simulink model "ipad2"  (Simulink 7.8)
settings: Solver=ode23tb  StartTime=0.0  StopTime=0.2  RelTol=1e-4
libraries: powerlib x97, powerlib_extras x1
settings Model: Creator=srujana  LastModifiedBy=srujana
settings SolverCC: MaxConsecutiveMinStep=auto  SolverResetMethod=Robust

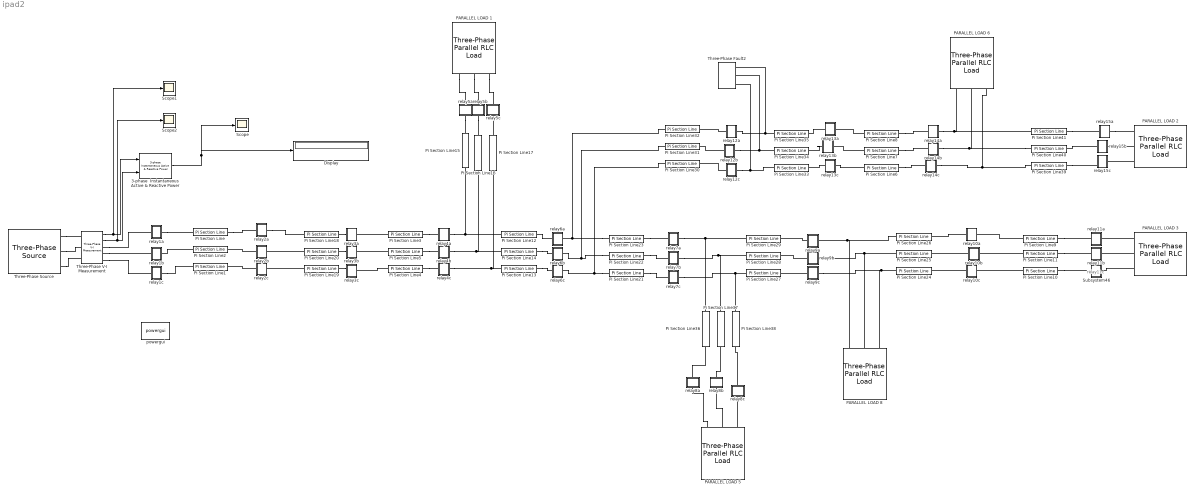
== system ipad2 ==
  note: relay11c
  3-phase  Instantaneous  Active & Reactive Power : powerlib_extras/Measurements/3-phase  Instantaneous  Active & Reactive Power
  Display : Display
      settings: Format=decimal (Stored Integer)
  PARALLEL LOAD 1 : powerlib/Elements/Three-Phase Parallel RLC Load  LConnTagsString=A|B|C  Configuration=Y (grounded)  NominalVoltage=10.27e3  NominalFrequency=50  ActivePower=1.85e6  InductivePower=1.28e6  CapacitivePower=0  Measurements=None  LoadType=constant Z
  PARALLEL LOAD 2 : powerlib/Elements/Three-Phase Parallel RLC Load  LConnTagsString=A|B|C  Configuration=Y (grounded)  NominalVoltage=10.27e3  NominalFrequency=50  ActivePower=0.91e6  InductivePower=0.63518e6  CapacitivePower=0  Measurements=None  LoadType=constant Z
  PARALLEL LOAD 3 : powerlib/Elements/Three-Phase Parallel RLC Load  LConnTagsString=A|B|C  Configuration=Y (grounded)  NominalVoltage=10.27e3  NominalFrequency=50  ActivePower=0.857e6  InductivePower=0.598e6  CapacitivePower=0  Measurements=None  LoadType=constant Z
  PARALLEL LOAD 5 : powerlib/Elements/Three-Phase Parallel RLC Load  LConnTagsString=A|B|C  Configuration=Y (grounded)  NominalVoltage=10.27e3  NominalFrequency=50  ActivePower=0.901e6  InductivePower=0.58046e6  CapacitivePower=0  Measurements=None  LoadType=constant Z
  PARALLEL LOAD 6 : powerlib/Elements/Three-Phase Parallel RLC Load  LConnTagsString=A|B|C  Configuration=Y (grounded)  NominalVoltage=10.27e3  NominalFrequency=50  ActivePower=0.92e6  InductivePower=0.64213e6  CapacitivePower=0  Measurements=None  LoadType=constant Z
  PARALLEL LOAD 8 : powerlib/Elements/Three-Phase Parallel RLC Load  LConnTagsString=A|B|C  Configuration=Y (grounded)  NominalVoltage=10.27e3  NominalFrequency=50  ActivePower=0.9e6  InductivePower=1.09756e6  CapacitivePower=0  Measurements=None  LoadType=constant Z
  Pi Section Line : powerlib/Elements/Pi Section Line  LConnTagsString=__new0  RConnTagsString=__new0  Frequency=50  Resistance=0.163  Inductance=0.28329e-3  Capacitance=445.633e-9  Length=0.078  PiSections=1  Measurements=None
      settings: AttributesFormatString=\n
  Pi Section Line1 : powerlib/Elements/Pi Section Line  LConnTagsString=__new0  RConnTagsString=__new0  Frequency=50  Resistance=0.163  Inductance=0.28329e-3  Capacitance=445.633e-9  Length=0.078  PiSections=1  Measurements=None
      settings: AttributesFormatString=\n
  Pi Section Line10 : powerlib/Elements/Pi Section Line  LConnTagsString=__new0  RConnTagsString=__new0  Frequency=50  Resistance=1.113  Inductance=0.37242e-3  Capacitance=190.985e-9  Length=0.1  PiSections=1  Measurements=None
      settings: AttributesFormatString=\n
  Pi Section Line11 : powerlib/Elements/Pi Section Line  LConnTagsString=__new0  RConnTagsString=__new0  Frequency=50  Resistance=1.113  Inductance=0.37242e-3  Capacitance=190.985e-9  Length=0.1  PiSections=1  Measurements=None
      settings: AttributesFormatString=\n
  Pi Section Line12 : powerlib/Elements/Pi Section Line  LConnTagsString=__new0  RConnTagsString=__new0  Frequency=50  Resistance=0.569  Inductance=0.3374e-3  Capacitance=254.647e-9  Length=0.33  PiSections=1  Measurements=None
      settings: AttributesFormatString=\n
  Pi Section Line13 : powerlib/Elements/Pi Section Line  LConnTagsString=__new0  RConnTagsString=__new0  Frequency=50  Resistance=0.569  Inductance=0.3374e-3  Capacitance=254.647e-9  Length=0.33  PiSections=1  Measurements=None
      settings: AttributesFormatString=\n
  Pi Section Line14 : powerlib/Elements/Pi Section Line  LConnTagsString=__new0  RConnTagsString=__new0  Frequency=50  Resistance=0.569  Inductance=0.3374e-3  Capacitance=254.647e-9  Length=0.33  PiSections=1  Measurements=None
      settings: AttributesFormatString=\n
  Pi Section Line15 : powerlib/Elements/Pi Section Line  LConnTagsString=__new0  RConnTagsString=__new0  Frequency=50  Resistance=0.569  Inductance=0.3374e-3  Capacitance=254.647e-9  Length=0.05  PiSections=1  Measurements=None
      settings: AttributesFormatString=\n
  Pi Section Line16 : powerlib/Elements/Pi Section Line  LConnTagsString=__new0  RConnTagsString=__new0  Frequency=50  Resistance=0.569  Inductance=0.3374e-3  Capacitance=254.647e-9  Length=0.05  PiSections=1  Measurements=None
      settings: AttributesFormatString=\n
  Pi Section Line17 : powerlib/Elements/Pi Section Line  LConnTagsString=__new0  RConnTagsString=__new0  Frequency=50  Resistance=0.569  Inductance=0.3374e-3  Capacitance=254.647e-9  Length=0.05  PiSections=1  Measurements=None
      settings: AttributesFormatString=\n
  Pi Section Line18 : powerlib/Elements/Pi Section Line  LConnTagsString=__new0  RConnTagsString=__new0  Frequency=50  Resistance=0.266  Inductance=0.30239e-3  Capacitance=318.309e-9  Length=0.85  PiSections=1  Measurements=None
      settings: AttributesFormatString=\n
  Pi Section Line19 : powerlib/Elements/Pi Section Line  LConnTagsString=__new0  RConnTagsString=__new0  Frequency=50  Resistance=0.266  Inductance=0.30239e-3  Capacitance=318.309e-9  Length=0.85  PiSections=1  Measurements=None
      settings: AttributesFormatString=\n
  Pi Section Line2 : powerlib/Elements/Pi Section Line  LConnTagsString=__new0  RConnTagsString=__new0  Frequency=50  Resistance=0.163  Inductance=0.28329e-3  Capacitance=445.633e-9  Length=0.078  PiSections=1  Measurements=None
      settings: AttributesFormatString=\n
  Pi Section Line20 : powerlib/Elements/Pi Section Line  LConnTagsString=__new0  RConnTagsString=__new0  Frequency=50  Resistance=0.266  Inductance=0.30239e-3  Capacitance=318.309e-9  Length=0.85  PiSections=1  Measurements=None
      settings: AttributesFormatString=\n
  Pi Section Line21 : powerlib/Elements/Pi Section Line  LConnTagsString=__new0  RConnTagsString=__new0  Frequency=50  Resistance=0.569  Inductance=0.3374e-3  Capacitance=254.647e-9  Length=0.2  PiSections=1  Measurements=None
      settings: AttributesFormatString=\n
  Pi Section Line22 : powerlib/Elements/Pi Section Line  LConnTagsString=__new0  RConnTagsString=__new0  Frequency=50  Resistance=0.569  Inductance=0.3374e-3  Capacitance=254.647e-9  Length=0.2  PiSections=1  Measurements=None
      settings: AttributesFormatString=\n
  Pi Section Line23 : powerlib/Elements/Pi Section Line  LConnTagsString=__new0  RConnTagsString=__new0  Frequency=50  Resistance=0.569  Inductance=0.3374e-3  Capacitance=254.647e-9  Length=0.2  PiSections=1  Measurements=None
      settings: AttributesFormatString=\n
  Pi Section Line24 : powerlib/Elements/Pi Section Line  LConnTagsString=__new0  RConnTagsString=__new0  Frequency=50  Resistance=0.569  Inductance=0.3374e-3  Capacitance=254.647e-9  Length=0.15  PiSections=1  Measurements=None
      settings: AttributesFormatString=\n
  Pi Section Line25 : powerlib/Elements/Pi Section Line  LConnTagsString=__new0  RConnTagsString=__new0  Frequency=50  Resistance=0.569  Inductance=0.3374e-3  Capacitance=254.647e-9  Length=0.15  PiSections=1  Measurements=None
      settings: AttributesFormatString=\n
  Pi Section Line26 : powerlib/Elements/Pi Section Line  LConnTagsString=__new0  RConnTagsString=__new0  Frequency=50  Resistance=0.569  Inductance=0.3374e-3  Capacitance=254.647e-9  Length=0.15  PiSections=1  Measurements=None
      settings: AttributesFormatString=\n
  Pi Section Line27 : powerlib/Elements/Pi Section Line  LConnTagsString=__new0  RConnTagsString=__new0  Frequency=50  Resistance=0.266  Inductance=0.30239e-3  Capacitance=318.309e-9  Length=0.65  PiSections=1  Measurements=None
      settings: AttributesFormatString=\n
  Pi Section Line28 : powerlib/Elements/Pi Section Line  LConnTagsString=__new0  RConnTagsString=__new0  Frequency=50  Resistance=0.266  Inductance=0.30239e-3  Capacitance=318.309e-9  Length=0.65  PiSections=1  Measurements=None
      settings: AttributesFormatString=\n
  Pi Section Line29 : powerlib/Elements/Pi Section Line  LConnTagsString=__new0  RConnTagsString=__new0  Frequency=50  Resistance=0.266  Inductance=0.30239e-3  Capacitance=318.309e-9  Length=0.65  PiSections=1  Measurements=None
      settings: AttributesFormatString=\n
  Pi Section Line3 : powerlib/Elements/Pi Section Line  LConnTagsString=__new0  RConnTagsString=__new0  Frequency=50  Resistance=0.569  Inductance=0.3374e-3  Capacitance=254.647e-9  Length=0.22  PiSections=1  Measurements=None
      settings: AttributesFormatString=\n
  Pi Section Line30 : powerlib/Elements/Pi Section Line  LConnTagsString=__new0  RConnTagsString=__new0  Frequency=50  Resistance=0.569  Inductance=0.3374e-3  Capacitance=254.647e-9  Length=0.44  PiSections=1  Measurements=None
      settings: AttributesFormatString=\n
  Pi Section Line31 : powerlib/Elements/Pi Section Line  LConnTagsString=__new0  RConnTagsString=__new0  Frequency=50  Resistance=0.569  Inductance=0.3374e-3  Capacitance=254.647e-9  Length=0.44  PiSections=1  Measurements=None
      settings: AttributesFormatString=\n
  Pi Section Line32 : powerlib/Elements/Pi Section Line  LConnTagsString=__new0  RConnTagsString=__new0  Frequency=50  Resistance=0.569  Inductance=0.3374e-3  Capacitance=254.647e-9  Length=0.44  PiSections=1  Measurements=None
      settings: AttributesFormatString=\n
  Pi Section Line33 : powerlib/Elements/Pi Section Line  LConnTagsString=__new0  RConnTagsString=__new0  Frequency=50  Resistance=0.266  Inductance=0.30239e-3  Capacitance=318.309e-9  Length=0.15  PiSections=1  Measurements=None
      settings: AttributesFormatString=\n
  Pi Section Line34 : powerlib/Elements/Pi Section Line  LConnTagsString=__new0  RConnTagsString=__new0  Frequency=50  Resistance=0.266  Inductance=0.30239e-3  Capacitance=318.309e-9  Length=0.15  PiSections=1  Measurements=None
      settings: AttributesFormatString=\n
  Pi Section Line35 : powerlib/Elements/Pi Section Line  LConnTagsString=__new0  RConnTagsString=__new0  Frequency=50  Resistance=0.266  Inductance=0.30239e-3  Capacitance=318.309e-9  Length=0.15  PiSections=1  Measurements=None
      settings: AttributesFormatString=\n
  Pi Section Line36 : powerlib/Elements/Pi Section Line  LConnTagsString=__new0  RConnTagsString=__new0  Frequency=50  Resistance=0.569  Inductance=0.3374e-3  Capacitance=254.647e-9  Length=0.04  PiSections=1  Measurements=None
      settings: AttributesFormatString=\n
  Pi Section Line37 : powerlib/Elements/Pi Section Line  LConnTagsString=__new0  RConnTagsString=__new0  Frequency=50  Resistance=0.569  Inductance=0.3374e-3  Capacitance=254.647e-9  Length=0.04  PiSections=1  Measurements=None
      settings: AttributesFormatString=\n
  Pi Section Line38 : powerlib/Elements/Pi Section Line  LConnTagsString=__new0  RConnTagsString=__new0  Frequency=50  Resistance=0.569  Inductance=0.3374e-3  Capacitance=254.647e-9  Length=0.04  PiSections=1  Measurements=None
      settings: AttributesFormatString=\n
  Pi Section Line39 : powerlib/Elements/Pi Section Line  LConnTagsString=__new0  RConnTagsString=__new0  Frequency=50  Resistance=0.266  Inductance=0.30239e-3  Capacitance=318.309e-9  Length=0.2  PiSections=1  Measurements=None
      settings: AttributesFormatString=\n
  Pi Section Line4 : powerlib/Elements/Pi Section Line  LConnTagsString=__new0  RConnTagsString=__new0  Frequency=50  Resistance=0.569  Inductance=0.3374e-3  Capacitance=254.647e-9  Length=0.22  PiSections=1  Measurements=None
      settings: AttributesFormatString=\n
  Pi Section Line40 : powerlib/Elements/Pi Section Line  LConnTagsString=__new0  RConnTagsString=__new0  Frequency=50  Resistance=0.266  Inductance=.30239e-3  Capacitance=318.309e-9  Length=0.2  PiSections=1  Measurements=None
      settings: AttributesFormatString=\n
  Pi Section Line41 : powerlib/Elements/Pi Section Line  LConnTagsString=__new0  RConnTagsString=__new0  Frequency=50  Resistance=0.266  Inductance=0.30239e-3  Capacitance=318.309e-9  Length=0.2  PiSections=1  Measurements=None
      settings: AttributesFormatString=\n
  Pi Section Line5 : powerlib/Elements/Pi Section Line  LConnTagsString=__new0  RConnTagsString=__new0  Frequency=50  Resistance=0.569  Inductance=0.3374e-3  Capacitance=254.647e-9  Length=0.22  PiSections=1  Measurements=None
      settings: AttributesFormatString=\n
  Pi Section Line6 : powerlib/Elements/Pi Section Line  LConnTagsString=__new0  RConnTagsString=__new0  Frequency=50  Resistance=0.266  Inductance=.30239e-3  Capacitance=318.309e-9  Length=0.45  PiSections=1  Measurements=None
      settings: AttributesFormatString=\n
  Pi Section Line7 : powerlib/Elements/Pi Section Line  LConnTagsString=__new0  RConnTagsString=__new0  Frequency=50  Resistance=0.266  Inductance=0.30239e-3  Capacitance=318.309e-9  Length=0.45  PiSections=1  Measurements=None
      settings: AttributesFormatString=\n
  Pi Section Line8 : powerlib/Elements/Pi Section Line  LConnTagsString=__new0  RConnTagsString=__new0  Frequency=50  Resistance=0.266  Inductance=0.30239e-3  Capacitance=318.309e-9  Length=0.45  PiSections=1  Measurements=None
      settings: AttributesFormatString=\n
  Pi Section Line9 : powerlib/Elements/Pi Section Line  LConnTagsString=__new0  RConnTagsString=__new0  Frequency=50  Resistance=1.113  Inductance=0.37242e-3  Capacitance=190.985e-9  Length=0.1  PiSections=1  Measurements=None
      settings: AttributesFormatString=\n
  Scope : Scope
      settings: YMin=3.9e+006  YMax=5.4e+006  SaveName=ScopeData46
  Scope1 : Scope
      settings: YMin=-700  YMax=600  SaveName=ScopeData47
  Scope2 : Scope
      settings: YMin=-700  YMax=600  SaveName=ScopeData48
  Subsystem46 : Subsystem
  Three-Phase V-I Measurement : powerlib/Measurements/Three-Phase V-I Measurement  VoltageMeasurement=phase-to-ground  SetLabelV=off  LabelV=Vabc  Vpu=off  VpuLL=off  CurrentMeasurement=yes  SetLabelI=off  LabelI=Iabc  Ipu=off  Pbase=100e6  Vbase=500e3  OutputType=Complex  PhasorSimulation=off  PSBequivalent=0
  Three-Phase Fault2 : powerlib/Elements/Three-Phase Fault  FaultA=on  FaultB=on  FaultC=on  FaultResistance=0.001  GroundFault=off  GroundResistance=0.001  External=off  SwitchStatus=[1 0]  SwitchTimes=[ 5/50 50/50]  InitialStates=[0 0 1]  SnubberResistance=1e6  SnubberCapacitance=inf  Measurements=Fault currents
  Three-Phase Source : powerlib/Electrical Sources/Three-Phase Source  Voltage=10.27e3  PhaseAngle=0  Frequency=50  InternalConnection=Yg  SpecifyImpedance=off  Resistance=0.00893  Inductance=16.52e-5  ShortCircuitLevel=100e6  BaseVoltage=10.27e3  XRratio=7  BusType=swing  Pref=0  Qref=0  Qmin=-inf  Qmax=inf
  powergui : powerlib/powergui  Priority=1  SimulationMode=Continuous  SolverType=Tustin  SampleTime=1/1600  frequency=60  SPID=off  DisableSnubberDevices=off  DisableRonSwitches=off  DisableVfSwitches=off  SwTol=0  Interpol=off  DisplayEquations=off  FunctionMessages=off  frequencyindice=0  Pbase=100e6  ErrMax=1e-4  Iterations=50  UnitsV=kV  UnitsW=MW  echomessages=off  HookPort=off  EnableUseOfTLC=off  x0status=blocks  RestoreLinks=warning  ResistiveCurrentMeasurement=off  Ylog=off  Xlog=on  ShowGrid=off  save=off  variable=ZData  ZoomFFT=off  StartTime=0.0  cycles=1  DisplayStyle=1  FreqAxis=off  MaxFrequency=1000  frequencyindicesteady=1  display=off  methode=off
  relay10a : Subsystem
  relay10b : Subsystem
  relay10c : Subsystem
  relay11a : Subsystem
  relay11b : Subsystem
  relay12a : Subsystem
  relay12b : Subsystem
  relay12c : Subsystem
  relay13a : Subsystem
  relay13b : Subsystem
  relay13c : Subsystem
  relay14a : Subsystem
  relay14b : Subsystem
  relay14c : Subsystem
  relay15a : Subsystem
  relay15b : Subsystem
  relay15c : Subsystem
  relay1a : Subsystem
  relay1b : Subsystem
  relay1c : Subsystem
  relay2a : Subsystem
  relay2b : Subsystem
  relay2c : Subsystem
  relay3a : Subsystem
  relay3b : Subsystem
  relay3c : Subsystem
  relay4a : Subsystem
  relay4b : Subsystem
  relay4c : Subsystem
  relay5a : Subsystem
  relay5b : Subsystem
  relay5c : Subsystem
  relay6a : Subsystem
  relay6b : Subsystem
  relay6c : Subsystem
  relay7a : Subsystem
  relay7b : Subsystem
  relay7c : Subsystem
  relay8a : Subsystem
  relay8b : Subsystem
  relay8c : Subsystem
  relay9a : Subsystem
  relay9b : Subsystem
  relay9c : Subsystem
  wires:
  Three-Phase V-I Measurement/1 -> 3-phase  Instantaneous  Active & Reactive Power/1, Scope1/1
  Three-Phase V-I Measurement/2 -> 3-phase  Instantaneous  Active & Reactive Power/2, Scope2/1
  3-phase  Instantaneous  Active & Reactive Power/1 -> Scope/1, Display/1
  connections:
  Pi Section Line18/RConn1 -- relay3a/LConn1
  Pi Section Line3/LConn1 -- relay3a/RConn1
  Pi Section Line20/RConn1 -- relay3b/LConn1
  Pi Section Line5/LConn1 -- relay3b/RConn1
  Pi Section Line19/RConn1 -- relay3c/LConn1
  Pi Section Line4/LConn1 -- relay3c/RConn1
  relay12a/LConn1 -- Pi Section Line32/RConn1
  relay12a/RConn1 -- Pi Section Line35/LConn1 -- Three-Phase Fault2/LConn1
  relay12b/LConn1 -- Pi Section Line31/RConn1
  relay12b/RConn1 -- Pi Section Line34/LConn1 -- Three-Phase Fault2/LConn2
  relay12c/LConn1 -- Pi Section Line30/RConn1
  relay12c/RConn1 -- Pi Section Line33/LConn1 -- Three-Phase Fault2/LConn3
  relay13c/LConn1 -- Pi Section Line33/RConn1
  relay13c/RConn1 -- Pi Section Line6/LConn1
  relay13b/LConn1 -- Pi Section Line34/RConn1
  Pi Section Line7/LConn1 -- relay13b/RConn1
  relay13a/LConn1 -- Pi Section Line35/RConn1
  Pi Section Line8/LConn1 -- relay13a/RConn1
  Pi Section Line3/RConn1 -- relay4a/LConn1
  relay4a/RConn1 -- Pi Section Line15/LConn1 -- Pi Section Line12/LConn1
  relay4c/RConn1 -- Pi Section Line13/LConn1 -- Pi Section Line17/LConn1
  Pi Section Line12/RConn1 -- relay6a/LConn1
  Pi Section Line14/RConn1 -- relay6b/LConn1
  Pi Section Line23/LConn1 -- relay6a/RConn1 -- Pi Section Line32/LConn1
  Pi Section Line22/LConn1 -- relay6b/RConn1 -- Pi Section Line31/LConn1
  Pi Section Line21/LConn1 -- relay6c/RConn1 -- Pi Section Line30/LConn1
  Pi Section Line23/RConn1 -- relay7a/LConn1
  Pi Section Line29/LConn1 -- Pi Section Line36/LConn1 -- relay7a/RConn1
  Pi Section Line22/RConn1 -- relay7b/LConn1
  relay7b/RConn1 -- Pi Section Line28/LConn1 -- Pi Section Line37/LConn1
  Pi Section Line21/RConn1 -- relay7c/LConn1
  relay7c/RConn1 -- Pi Section Line27/LConn1 -- Pi Section Line38/LConn1
  Pi Section Line8/RConn1 -- relay14a/LConn1
  Pi Section Line7/RConn1 -- relay14b/LConn1
  Pi Section Line6/RConn1 -- relay14c/LConn1
  Pi Section Line41/LConn1 -- PARALLEL LOAD 6/LConn1 -- relay14a/RConn1
  Pi Section Line40/LConn1 -- PARALLEL LOAD 6/LConn2 -- relay14b/RConn1
  Pi Section Line39/LConn1 -- PARALLEL LOAD 6/LConn3 -- relay14c/RConn1
  relay10b/LConn1 -- Pi Section Line25/RConn1
  Pi Section Line11/LConn1 -- relay10b/RConn1
  relay10c/LConn1 -- Pi Section Line24/RConn1
  Pi Section Line10/LConn1 -- relay10c/RConn1
  PARALLEL LOAD 1/LConn1 -- relay5a/LConn1
  PARALLEL LOAD 1/LConn2 -- relay5b/LConn1
  PARALLEL LOAD 1/LConn3 -- relay5c/LConn1
  relay5a/RConn1 -- Pi Section Line15/RConn1
  relay5b/RConn1 -- Pi Section Line16/RConn1
  relay5c/RConn1 -- Pi Section Line17/RConn1
  relay4b/RConn1 -- Pi Section Line16/LConn1 -- Pi Section Line14/LConn1
  Pi Section Line9/RConn1 -- relay11a/LConn1
  Pi Section Line11/RConn1 -- relay11b/LConn1
  Pi Section Line10/RConn1 -- Subsystem46/LConn1
  PARALLEL LOAD 3/LConn1 -- relay11a/RConn1
  PARALLEL LOAD 3/LConn2 -- relay11b/RConn1
  PARALLEL LOAD 3/LConn3 -- Subsystem46/RConn1
  relay8a/RConn1 -- Pi Section Line36/RConn1
  relay8b/RConn1 -- Pi Section Line37/RConn1
  relay8c/RConn1 -- Pi Section Line38/RConn1
  relay8a/LConn1 -- PARALLEL LOAD 5/LConn1
  relay8b/LConn1 -- PARALLEL LOAD 5/LConn2
  relay8c/LConn1 -- PARALLEL LOAD 5/LConn3
  Pi Section Line41/RConn1 -- relay15a/LConn1
  Pi Section Line40/RConn1 -- relay15b/LConn1
  Pi Section Line39/RConn1 -- relay15c/LConn1
  relay15a/RConn1 -- PARALLEL LOAD 2/LConn1
  PARALLEL LOAD 2/LConn2 -- relay15b/RConn1
  PARALLEL LOAD 2/LConn3 -- relay15c/RConn1
  relay9a/LConn1 -- Pi Section Line29/RConn1
  relay9b/LConn1 -- Pi Section Line28/RConn1
  relay9c/LConn1 -- Pi Section Line27/RConn1
  relay9b/RConn1 -- Pi Section Line25/LConn1 -- PARALLEL LOAD 8/LConn2
  relay9c/RConn1 -- Pi Section Line24/LConn1 -- PARALLEL LOAD 8/LConn3
  Pi Section Line5/RConn1 -- relay4b/LConn1
  Pi Section Line4/RConn1 -- relay4c/LConn1
  relay1a/RConn1 -- Pi Section Line/LConn1
  relay1b/RConn1 -- Pi Section Line2/LConn1
  relay1c/RConn1 -- Pi Section Line1/LConn1
  Pi Section Line/RConn1 -- relay2a/LConn1
  relay2a/RConn1 -- Pi Section Line18/LConn1
  relay2b/LConn1 -- Pi Section Line2/RConn1
  Pi Section Line20/LConn1 -- relay2b/RConn1
  relay2c/LConn1 -- Pi Section Line1/RConn1
  Pi Section Line19/LConn1 -- relay2c/RConn1
  Pi Section Line13/RConn1 -- relay6c/LConn1
  Three-Phase Source/RConn1 -- Three-Phase V-I Measurement/LConn1
  Three-Phase Source/RConn2 -- Three-Phase V-I Measurement/LConn2
  Three-Phase Source/RConn3 -- Three-Phase V-I Measurement/LConn3
  Three-Phase V-I Measurement/RConn1 -- relay1a/LConn1
  Three-Phase V-I Measurement/RConn2 -- relay1b/LConn1
  Three-Phase V-I Measurement/RConn3 -- relay1c/LConn1
  Pi Section Line9/LConn1 -- relay10a/RConn1
  relay10a/LConn1 -- Pi Section Line26/RConn1
  relay9a/RConn1 -- Pi Section Line26/LConn1 -- PARALLEL LOAD 8/LConn1

== system ipad2/Subsystem46 ==
  Current Measurement : powerlib/Measurements/Current Measurement  PhasorSimulation=off  OutputType=Complex  PSBequivalent=0
  Scope : Scope
      settings: SaveName=ScopeData31
  ic11 : ToWorkspace  VariableName=ic11  SampleTime=1/1600  SaveFormat=Array
  Conn1 : PMIOPort  Port=1  Side=Left
  Conn2 : PMIOPort  Port=2  Side=Right
  wires:
  Current Measurement/1 -> ic11/1, Scope/1
  connections:
  Conn2/RConn1 -- Current Measurement/RConn1
  Conn1/RConn1 -- Current Measurement/LConn1

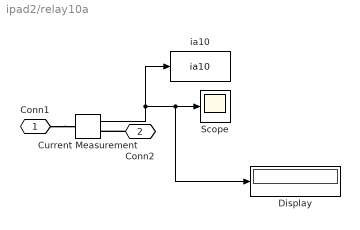
== system ipad2/relay10a ==
  Current Measurement : powerlib/Measurements/Current Measurement  PhasorSimulation=off  OutputType=Complex  PSBequivalent=0
  Display : Display
  Scope : Scope
      settings: TimeRange=0.004000000000000004  YMin=-80  YMax=-40  SaveName=ScopeData26
  ia10 : ToWorkspace  VariableName=ia10  SampleTime=1/1600  SaveFormat=Array
  Conn1 : PMIOPort  Port=1  Side=Left
  Conn2 : PMIOPort  Port=2  Side=Right
  wires:
  Current Measurement/1 -> ia10/1, Scope/1, Display/1
  connections:
  Conn1/RConn1 -- Current Measurement/LConn1
  Conn2/RConn1 -- Current Measurement/RConn1

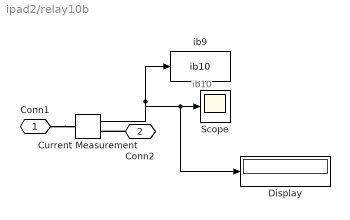
== system ipad2/relay10b ==
  note: ib10
  Current Measurement : powerlib/Measurements/Current Measurement  PhasorSimulation=off  OutputType=Complex  PSBequivalent=0
  Display : Display
  Scope : Scope
      settings: SaveName=ScopeData27
  ib9 : ToWorkspace  VariableName=ib10  SampleTime=1/1600  SaveFormat=Array
  Conn1 : PMIOPort  Port=1  Side=Left
  Conn2 : PMIOPort  Port=2  Side=Right
  wires:
  Current Measurement/1 -> ib9/1, Scope/1, Display/1
  connections:
  Conn2/RConn1 -- Current Measurement/RConn1
  Conn1/RConn1 -- Current Measurement/LConn1

== system ipad2/relay10c ==
  Current Measurement : powerlib/Measurements/Current Measurement  PhasorSimulation=off  OutputType=Complex  PSBequivalent=0
  Scope : Scope
      settings: SaveName=ScopeData28
  ic10 : ToWorkspace  VariableName=ic10  SampleTime=1/1600  SaveFormat=Array
  Conn1 : PMIOPort  Port=1  Side=Left
  Conn2 : PMIOPort  Port=2  Side=Right
  wires:
  Current Measurement/1 -> ic10/1, Scope/1
  connections:
  Conn2/RConn1 -- Current Measurement/RConn1
  Conn1/RConn1 -- Current Measurement/LConn1

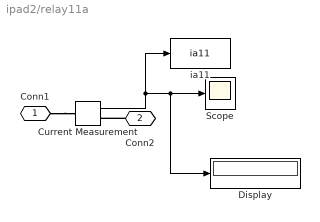
== system ipad2/relay11a ==
  Current Measurement : powerlib/Measurements/Current Measurement  PhasorSimulation=off  OutputType=Complex  PSBequivalent=0
  Display : Display
  Scope : Scope
      settings: SaveName=ScopeData29
  ia11 : ToWorkspace  VariableName=ia11  SampleTime=1/1600  SaveFormat=Array
  Conn1 : PMIOPort  Port=1  Side=Left
  Conn2 : PMIOPort  Port=2  Side=Right
  wires:
  Current Measurement/1 -> ia11/1, Scope/1, Display/1
  connections:
  Conn2/RConn1 -- Current Measurement/RConn1
  Conn1/RConn1 -- Current Measurement/LConn1

== system ipad2/relay11b ==
  Current Measurement : powerlib/Measurements/Current Measurement  PhasorSimulation=off  OutputType=Complex  PSBequivalent=0
  Scope : Scope
      settings: SaveName=ScopeData30
  ib11 : ToWorkspace  VariableName=ib11  SampleTime=1/1600  SaveFormat=Array
  Conn1 : PMIOPort  Port=1  Side=Left
  Conn2 : PMIOPort  Port=2  Side=Right
  wires:
  Current Measurement/1 -> ib11/1, Scope/1
  connections:
  Conn1/RConn1 -- Current Measurement/LConn1
  Conn2/RConn1 -- Current Measurement/RConn1

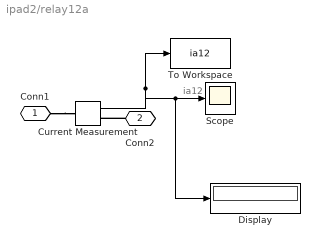
== system ipad2/relay12a ==
  note: ia12
  Current Measurement : powerlib/Measurements/Current Measurement  PhasorSimulation=off  OutputType=Complex  PSBequivalent=0
  Display : Display
  Scope : Scope
      settings: SaveName=ScopeData32
  To Workspace : ToWorkspace  VariableName=ia12  SampleTime=1/1600  SaveFormat=Array
  Conn1 : PMIOPort  Port=1  Side=Left
  Conn2 : PMIOPort  Port=2  Side=Right
  wires:
  Current Measurement/1 -> To Workspace/1, Scope/1, Display/1
  connections:
  Conn1/RConn1 -- Current Measurement/LConn1
  Conn2/RConn1 -- Current Measurement/RConn1

== system ipad2/relay12b ==
  Current Measurement : powerlib/Measurements/Current Measurement  PhasorSimulation=off  OutputType=Complex  PSBequivalent=0
  Scope : Scope
      settings: SaveName=ScopeData33
  ib12 : ToWorkspace  VariableName=ib12  SampleTime=1/1600  SaveFormat=Array
  Conn1 : PMIOPort  Port=1  Side=Left
  Conn2 : PMIOPort  Port=2  Side=Right
  wires:
  Current Measurement/1 -> ib12/1, Scope/1
  connections:
  Conn2/RConn1 -- Current Measurement/RConn1
  Conn1/RConn1 -- Current Measurement/LConn1

== system ipad2/relay12c ==
  note: ic12
  Current Measurement : powerlib/Measurements/Current Measurement  PhasorSimulation=off  OutputType=Complex  PSBequivalent=0
  Scope : Scope
      settings: SaveName=ScopeData34
  To Workspace : ToWorkspace  VariableName=ic12  SampleTime=1/1600  SaveFormat=Array
  Conn1 : PMIOPort  Port=1  Side=Left
  Conn2 : PMIOPort  Port=2  Side=Right
  wires:
  Current Measurement/1 -> To Workspace/1, Scope/1
  connections:
  Conn1/RConn1 -- Current Measurement/LConn1
  Conn2/RConn1 -- Current Measurement/RConn1

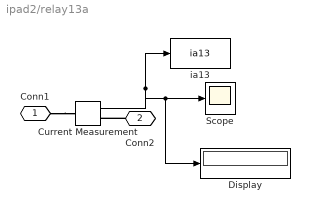
== system ipad2/relay13a ==
  Current Measurement : powerlib/Measurements/Current Measurement  PhasorSimulation=off  OutputType=Complex  PSBequivalent=0
  Display : Display
  Scope : Scope
      settings: SaveName=ScopeData35
  ia13 : ToWorkspace  VariableName=ia13  SampleTime=1/1660  SaveFormat=Array
  Conn1 : PMIOPort  Port=1  Side=Left
  Conn2 : PMIOPort  Port=2  Side=Right
  wires:
  Current Measurement/1 -> ia13/1, Scope/1, Display/1
  connections:
  Conn2/RConn1 -- Current Measurement/RConn1
  Conn1/RConn1 -- Current Measurement/LConn1

== system ipad2/relay13b ==
  Current Measurement : powerlib/Measurements/Current Measurement  PhasorSimulation=off  OutputType=Complex  PSBequivalent=0
  Scope : Scope
      settings: SaveName=ScopeData36
  ib13 : ToWorkspace  VariableName=ib13  SampleTime=1/1600  SaveFormat=Array
  Conn1 : PMIOPort  Port=1  Side=Left
  Conn2 : PMIOPort  Port=2  Side=Right
  wires:
  Current Measurement/1 -> ib13/1, Scope/1
  connections:
  Conn1/RConn1 -- Current Measurement/LConn1
  Conn2/RConn1 -- Current Measurement/RConn1

== system ipad2/relay13c ==
  Current Measurement : powerlib/Measurements/Current Measurement  PhasorSimulation=off  OutputType=Complex  PSBequivalent=0
  Scope : Scope
      settings: SaveName=ScopeData37
  ic13 : ToWorkspace  VariableName=ic13  SampleTime=1/1600  SaveFormat=Array
  Conn1 : PMIOPort  Port=1  Side=Left
  Conn2 : PMIOPort  Port=2  Side=Right
  wires:
  Current Measurement/1 -> ic13/1, Scope/1
  connections:
  Conn2/RConn1 -- Current Measurement/RConn1
  Conn1/RConn1 -- Current Measurement/LConn1

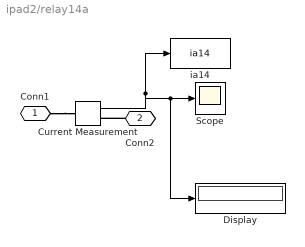
== system ipad2/relay14a ==
  Current Measurement : powerlib/Measurements/Current Measurement  PhasorSimulation=off  OutputType=Complex  PSBequivalent=0
  Display : Display
  Scope : Scope
      settings: SaveName=ScopeData38
  ia14 : ToWorkspace  VariableName=ia14  SampleTime=1/1600  SaveFormat=Array
  Conn1 : PMIOPort  Port=1  Side=Left
  Conn2 : PMIOPort  Port=2  Side=Right
  wires:
  Current Measurement/1 -> ia14/1, Scope/1, Display/1
  connections:
  Conn1/RConn1 -- Current Measurement/LConn1
  Conn2/RConn1 -- Current Measurement/RConn1

== system ipad2/relay14b ==
  Current Measurement : powerlib/Measurements/Current Measurement  PhasorSimulation=off  OutputType=Complex  PSBequivalent=0
  Scope : Scope
      settings: SaveName=ScopeData39
  ib14 : ToWorkspace  VariableName=ib14  SampleTime=1/1600  SaveFormat=Array
  Conn1 : PMIOPort  Port=1  Side=Left
  Conn2 : PMIOPort  Port=2  Side=Right
  wires:
  Current Measurement/1 -> ib14/1, Scope/1
  connections:
  Conn2/RConn1 -- Current Measurement/RConn1
  Conn1/RConn1 -- Current Measurement/LConn1

== system ipad2/relay14c ==
  Current Measurement : powerlib/Measurements/Current Measurement  PhasorSimulation=off  OutputType=Complex  PSBequivalent=0
  Scope : Scope
      settings: SaveName=ScopeData40
  ic14 : ToWorkspace  VariableName=ic14  SampleTime=1/1600  SaveFormat=Array
  Conn1 : PMIOPort  Port=1  Side=Left
  Conn2 : PMIOPort  Port=2  Side=Right
  wires:
  Current Measurement/1 -> ic14/1, Scope/1
  connections:
  Conn1/RConn1 -- Current Measurement/LConn1
  Conn2/RConn1 -- Current Measurement/RConn1

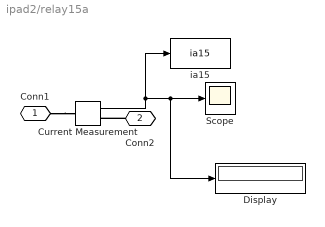
== system ipad2/relay15a ==
  Current Measurement : powerlib/Measurements/Current Measurement  PhasorSimulation=off  OutputType=Complex  PSBequivalent=0
  Display : Display
  Scope : Scope
      settings: SaveName=ScopeData41
  ia15 : ToWorkspace  VariableName=ia15  SampleTime=1/1600  SaveFormat=Array
  Conn1 : PMIOPort  Port=1  Side=Left
  Conn2 : PMIOPort  Port=2  Side=Right
  wires:
  Current Measurement/1 -> ia15/1, Scope/1, Display/1
  connections:
  Conn2/RConn1 -- Current Measurement/RConn1
  Conn1/RConn1 -- Current Measurement/LConn1

== system ipad2/relay15b ==
  note: ib15
  Current Measurement : powerlib/Measurements/Current Measurement  PhasorSimulation=off  OutputType=Complex  PSBequivalent=0
  Scope : Scope
      settings: SaveName=ScopeData42
  ib14 : ToWorkspace  VariableName=ib15  SampleTime=1/1600  SaveFormat=Array
  Conn1 : PMIOPort  Port=1  Side=Left
  Conn2 : PMIOPort  Port=2  Side=Right
  wires:
  Current Measurement/1 -> ib14/1, Scope/1
  connections:
  Conn1/RConn1 -- Current Measurement/LConn1
  Conn2/RConn1 -- Current Measurement/RConn1

== system ipad2/relay15c ==
  Current Measurement : powerlib/Measurements/Current Measurement  PhasorSimulation=off  OutputType=Complex  PSBequivalent=0
  Scope2 : Scope
      settings: SaveName=ScopeData45
  ic15 : ToWorkspace  VariableName=ic15  SampleTime=1/1600  SaveFormat=Array
  Conn1 : PMIOPort  Port=1  Side=Left
  Conn2 : PMIOPort  Port=2  Side=Right
  wires:
  Current Measurement/1 -> ic15/1, Scope2/1
  connections:
  Conn2/RConn1 -- Current Measurement/RConn1
  Conn1/RConn1 -- Current Measurement/LConn1

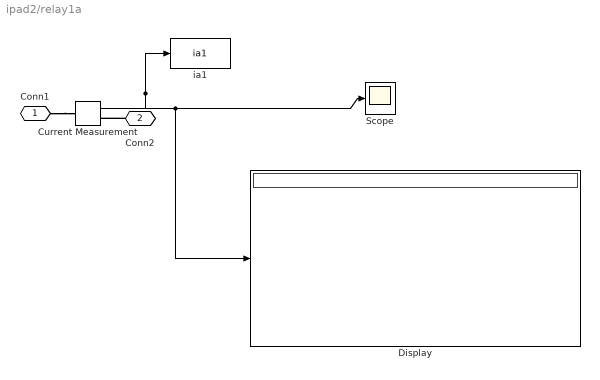
== system ipad2/relay1a ==
  Current Measurement : powerlib/Measurements/Current Measurement  PhasorSimulation=off  OutputType=Complex  PSBequivalent=0
  Display : Display
  Scope : Scope
      settings: YMin=-700  YMax=600
  ia1 : ToWorkspace  VariableName=ia1  SampleTime=1/1600  SaveFormat=Array
  Conn1 : PMIOPort  Port=1  Side=Left
  Conn2 : PMIOPort  Port=2  Side=Right
  wires:
  Current Measurement/1 -> ia1/1, Scope/1, Display/1
  connections:
  Conn2/RConn1 -- Current Measurement/RConn1
  Conn1/RConn1 -- Current Measurement/LConn1

== system ipad2/relay1b ==
  Current Measurement : powerlib/Measurements/Current Measurement  PhasorSimulation=off  OutputType=Complex  PSBequivalent=0
  Scope : Scope
  ib1 : ToWorkspace  VariableName=ib1  SampleTime=1/1600  SaveFormat=Array
  Conn1 : PMIOPort  Port=1  Side=Left
  Conn2 : PMIOPort  Port=2  Side=Right
  wires:
  Current Measurement/1 -> ib1/1, Scope/1
  connections:
  Conn1/RConn1 -- Current Measurement/LConn1
  Conn2/RConn1 -- Current Measurement/RConn1

== system ipad2/relay1c ==
  Current Measurement : powerlib/Measurements/Current Measurement  PhasorSimulation=off  OutputType=Complex  PSBequivalent=0
  Scope : Scope
      settings: SaveName=ScopeData2
  ic1 : ToWorkspace  VariableName=ic1  SampleTime=1/1600  SaveFormat=Array
  Conn1 : PMIOPort  Port=1  Side=Left
  Conn2 : PMIOPort  Port=2  Side=Right
  wires:
  Current Measurement/1 -> ic1/1, Scope/1
  connections:
  Conn2/RConn1 -- Current Measurement/RConn1
  Conn1/RConn1 -- Current Measurement/LConn1

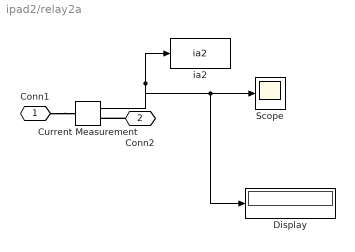
== system ipad2/relay2a ==
  Current Measurement : powerlib/Measurements/Current Measurement  PhasorSimulation=off  OutputType=Complex  PSBequivalent=0
  Display : Display
  Scope : Scope
      settings: YMin=-625  YMax=-275  SaveName=ScopeData3
  ia2 : ToWorkspace  VariableName=ia2  SampleTime=1/1600  SaveFormat=Array
  Conn1 : PMIOPort  Port=1  Side=Left
  Conn2 : PMIOPort  Port=2  Side=Right
  wires:
  Current Measurement/1 -> ia2/1, Scope/1, Display/1
  connections:
  Conn1/RConn1 -- Current Measurement/LConn1
  Conn2/RConn1 -- Current Measurement/RConn1

== system ipad2/relay2b ==
  Current Measurement : powerlib/Measurements/Current Measurement  PhasorSimulation=off  OutputType=Complex  PSBequivalent=0
  Scope : Scope
      settings: SaveName=ScopeData4
  ib2 : ToWorkspace  VariableName=ib2  SampleTime=1/1600  SaveFormat=Array
  Conn1 : PMIOPort  Port=1  Side=Left
  Conn2 : PMIOPort  Port=2  Side=Right
  wires:
  Current Measurement/1 -> ib2/1, Scope/1
  connections:
  Conn2/RConn1 -- Current Measurement/RConn1
  Conn1/RConn1 -- Current Measurement/LConn1

== system ipad2/relay2c ==
  Current Measurement : powerlib/Measurements/Current Measurement  PhasorSimulation=off  OutputType=Complex  PSBequivalent=0
  Scope : Scope
      settings: SaveName=ScopeData5
  ic2 : ToWorkspace  VariableName=ic2  SampleTime=1/1600  SaveFormat=Array
  Conn1 : PMIOPort  Port=1  Side=Left
  Conn2 : PMIOPort  Port=2  Side=Right
  wires:
  Current Measurement/1 -> ic2/1, Scope/1
  connections:
  Conn1/RConn1 -- Current Measurement/LConn1
  Conn2/RConn1 -- Current Measurement/RConn1

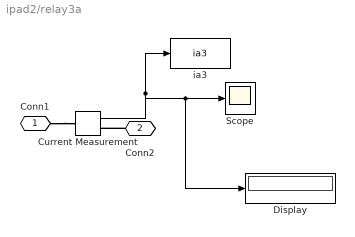
== system ipad2/relay3a ==
  Current Measurement : powerlib/Measurements/Current Measurement  PhasorSimulation=off  OutputType=Complex  PSBequivalent=0
  Display : Display
  Scope : Scope
      settings: SaveName=ScopeData6
  ia3 : ToWorkspace  VariableName=ia3  SampleTime=1/1600  SaveFormat=Array
  Conn1 : PMIOPort  Port=1  Side=Left
  Conn2 : PMIOPort  Port=2  Side=Right
  wires:
  Current Measurement/1 -> ia3/1, Scope/1, Display/1
  connections:
  Conn1/RConn1 -- Current Measurement/LConn1
  Conn2/RConn1 -- Current Measurement/RConn1

== system ipad2/relay3b ==
  Current Measurement : powerlib/Measurements/Current Measurement  PhasorSimulation=off  OutputType=Complex  PSBequivalent=0
  Scope : Scope
      settings: SaveName=ScopeData7
  ib3 : ToWorkspace  VariableName=ib3  SampleTime=1/1600  SaveFormat=Array
  Conn1 : PMIOPort  Port=1  Side=Left
  Conn2 : PMIOPort  Port=2  Side=Right
  wires:
  Current Measurement/1 -> ib3/1, Scope/1
  connections:
  Conn2/RConn1 -- Current Measurement/RConn1
  Conn1/RConn1 -- Current Measurement/LConn1

== system ipad2/relay3c ==
  Current Measurement : powerlib/Measurements/Current Measurement  PhasorSimulation=off  OutputType=Complex  PSBequivalent=0
  Scope : Scope
      settings: SaveName=ScopeData8
  ic3 : ToWorkspace  VariableName=ic3  SampleTime=1/1600  SaveFormat=Array
  Conn1 : PMIOPort  Port=1  Side=Left
  Conn2 : PMIOPort  Port=2  Side=Right
  wires:
  Current Measurement/1 -> ic3/1, Scope/1
  connections:
  Conn2/RConn1 -- Current Measurement/RConn1
  Conn1/RConn1 -- Current Measurement/LConn1

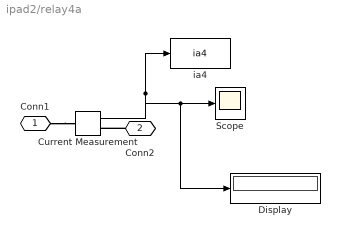
== system ipad2/relay4a ==
  Current Measurement : powerlib/Measurements/Current Measurement  PhasorSimulation=off  OutputType=Complex  PSBequivalent=0
  Display : Display
  Scope : Scope
      settings: SaveName=ScopeData9
  ia4 : ToWorkspace  VariableName=ia4  SampleTime=1/1600  SaveFormat=Array
  Conn1 : PMIOPort  Port=1  Side=Left
  Conn2 : PMIOPort  Port=2  Side=Right
  wires:
  Current Measurement/1 -> ia4/1, Scope/1, Display/1
  connections:
  Conn1/RConn1 -- Current Measurement/LConn1
  Conn2/RConn1 -- Current Measurement/RConn1

== system ipad2/relay4b ==
  Current Measurement : powerlib/Measurements/Current Measurement  PhasorSimulation=off  OutputType=Complex  PSBequivalent=0
  Scope : Scope
      settings: SaveName=ScopeData10
  ib4 : ToWorkspace  VariableName=ib4  SampleTime=1/1600  SaveFormat=Array
  Conn1 : PMIOPort  Port=1  Side=Left
  Conn2 : PMIOPort  Port=2  Side=Right
  wires:
  Current Measurement/1 -> ib4/1, Scope/1
  connections:
  Conn2/RConn1 -- Current Measurement/RConn1
  Conn1/RConn1 -- Current Measurement/LConn1

== system ipad2/relay4c ==
  Current Measurement : powerlib/Measurements/Current Measurement  PhasorSimulation=off  OutputType=Complex  PSBequivalent=0
  Scope : Scope
      settings: SaveName=ScopeData49
  ic4 : ToWorkspace  VariableName=ic4  SampleTime=1/1600  SaveFormat=Array
  Conn1 : PMIOPort  Port=1  Side=Left
  Conn2 : PMIOPort  Port=2  Side=Right
  wires:
  Current Measurement/1 -> ic4/1, Scope/1
  connections:
  Conn1/RConn1 -- Current Measurement/LConn1
  Conn2/RConn1 -- Current Measurement/RConn1

== system ipad2/relay5a ==
  Current Measurement : powerlib/Measurements/Current Measurement  PhasorSimulation=off  OutputType=Complex  PSBequivalent=0
  Display : Display
  Scope : Scope
      settings: SaveName=ScopeData11
  ia5 : ToWorkspace  VariableName=ia5  SampleTime=1/1600  SaveFormat=Array
  Conn1 : PMIOPort  Port=1  Side=Left
  Conn2 : PMIOPort  Port=2  Side=Right
  wires:
  Current Measurement/1 -> ia5/1, Scope/1, Display/1
  connections:
  Conn1/RConn1 -- Current Measurement/LConn1
  Conn2/RConn1 -- Current Measurement/RConn1

== system ipad2/relay5b ==
  Current Measurement : powerlib/Measurements/Current Measurement  PhasorSimulation=off  OutputType=Complex  PSBequivalent=0
  Scope : Scope
      settings: SaveName=ScopeData12
  ib5 : ToWorkspace  VariableName=ib5  SampleTime=1/1600  SaveFormat=Array
  Conn1 : PMIOPort  Port=1  Side=Left
  Conn2 : PMIOPort  Port=2  Side=Right
  wires:
  Current Measurement/1 -> ib5/1, Scope/1
  connections:
  Conn1/RConn1 -- Current Measurement/LConn1
  Conn2/RConn1 -- Current Measurement/RConn1

== system ipad2/relay5c ==
  Current Measurement : powerlib/Measurements/Current Measurement  PhasorSimulation=off  OutputType=Complex  PSBequivalent=0
  Scope : Scope
      settings: SaveName=ScopeData13
  ic5 : ToWorkspace  VariableName=ic5  SampleTime=1/1600  SaveFormat=Array
  Conn1 : PMIOPort  Port=1  Side=Left
  Conn2 : PMIOPort  Port=2  Side=Right
  wires:
  Current Measurement/1 -> ic5/1, Scope/1
  connections:
  Conn2/RConn1 -- Current Measurement/RConn1
  Conn1/RConn1 -- Current Measurement/LConn1

== system ipad2/relay6a ==
  Current Measurement : powerlib/Measurements/Current Measurement  PhasorSimulation=off  OutputType=Complex  PSBequivalent=0
  Display : Display
  Scope : Scope
      settings: SaveName=ScopeData14
  ia6 : ToWorkspace  VariableName=ia6  SampleTime=1/1600  SaveFormat=Array
  Conn1 : PMIOPort  Port=1  Side=Left
  Conn2 : PMIOPort  Port=2  Side=Right
  wires:
  Current Measurement/1 -> ia6/1, Scope/1, Display/1
  connections:
  Conn2/RConn1 -- Current Measurement/RConn1
  Conn1/RConn1 -- Current Measurement/LConn1

== system ipad2/relay6b ==
  Current Measurement : powerlib/Measurements/Current Measurement  PhasorSimulation=off  OutputType=Complex  PSBequivalent=0
  Scope : Scope
      settings: SaveName=ScopeData15
  ib6 : ToWorkspace  VariableName=ib6  SampleTime=1/1600  SaveFormat=Array
  Conn1 : PMIOPort  Port=1  Side=Left
  Conn2 : PMIOPort  Port=2  Side=Right
  wires:
  Current Measurement/1 -> ib6/1, Scope/1
  connections:
  Conn1/RConn1 -- Current Measurement/LConn1
  Conn2/RConn1 -- Current Measurement/RConn1

== system ipad2/relay6c ==
  note: ic6
  Current Measurement : powerlib/Measurements/Current Measurement  PhasorSimulation=off  OutputType=Complex  PSBequivalent=0
  Scope : Scope
      settings: SaveName=ScopeData16
  To Workspace : ToWorkspace  VariableName=ic6  SampleTime=1/1600  SaveFormat=Array
  Conn1 : PMIOPort  Port=1  Side=Left
  Conn2 : PMIOPort  Port=2  Side=Right
  wires:
  Current Measurement/1 -> To Workspace/1, Scope/1
  connections:
  Conn2/RConn1 -- Current Measurement/RConn1
  Conn1/RConn1 -- Current Measurement/LConn1

== system ipad2/relay7a ==
  Current Measurement : powerlib/Measurements/Current Measurement  PhasorSimulation=off  OutputType=Complex  PSBequivalent=0
  Display : Display
  Scope : Scope
      settings: SaveName=ScopeData17
  ia7 : ToWorkspace  VariableName=ia7  SampleTime=1/1600  SaveFormat=Array
  Conn1 : PMIOPort  Port=1  Side=Left
  Conn2 : PMIOPort  Port=2  Side=Right
  wires:
  Current Measurement/1 -> ia7/1, Scope/1, Display/1
  connections:
  Conn2/RConn1 -- Current Measurement/RConn1
  Conn1/RConn1 -- Current Measurement/LConn1

== system ipad2/relay7b ==
  Current Measurement : powerlib/Measurements/Current Measurement  PhasorSimulation=off  OutputType=Complex  PSBequivalent=0
  Scope : Scope
      settings: SaveName=ScopeData18
  ib7 : ToWorkspace  VariableName=ib7  SampleTime=1/1600  SaveFormat=Array
  Conn1 : PMIOPort  Port=1  Side=Left
  Conn2 : PMIOPort  Port=2  Side=Right
  wires:
  Current Measurement/1 -> ib7/1, Scope/1
  connections:
  Conn1/RConn1 -- Current Measurement/LConn1
  Conn2/RConn1 -- Current Measurement/RConn1

== system ipad2/relay7c ==
  Current Measurement : powerlib/Measurements/Current Measurement  PhasorSimulation=off  OutputType=Complex  PSBequivalent=0
  Scope : Scope
      settings: SaveName=ScopeData19
  ic7 : ToWorkspace  VariableName=ic7  SampleTime=1/1600  SaveFormat=Array
  Conn1 : PMIOPort  Port=1  Side=Left
  Conn2 : PMIOPort  Port=2  Side=Right
  wires:
  Current Measurement/1 -> ic7/1, Scope/1
  connections:
  Conn2/RConn1 -- Current Measurement/RConn1
  Conn1/RConn1 -- Current Measurement/LConn1

== system ipad2/relay8a ==
  Current Measurement : powerlib/Measurements/Current Measurement  PhasorSimulation=off  OutputType=Complex  PSBequivalent=0
  Display : Display
  Scope : Scope
      settings: SaveName=ScopeData20
  ia8 : ToWorkspace  VariableName=ia8  SampleTime=1/1600  SaveFormat=Array
  Conn1 : PMIOPort  Port=1  Side=Left
  Conn2 : PMIOPort  Port=2  Side=Right
  wires:
  Current Measurement/1 -> ia8/1, Scope/1, Display/1
  connections:
  Conn2/RConn1 -- Current Measurement/RConn1
  Conn1/RConn1 -- Current Measurement/LConn1

== system ipad2/relay8b ==
  Current Measurement : powerlib/Measurements/Current Measurement  PhasorSimulation=off  OutputType=Complex  PSBequivalent=0
  Scope : Scope
      settings: SaveName=ScopeData21
  ib8 : ToWorkspace  VariableName=ib8  SampleTime=1/1600  SaveFormat=Array
  Conn1 : PMIOPort  Port=1  Side=Left
  Conn2 : PMIOPort  Port=2  Side=Right
  wires:
  Current Measurement/1 -> ib8/1, Scope/1
  connections:
  Conn1/RConn1 -- Current Measurement/LConn1
  Conn2/RConn1 -- Current Measurement/RConn1

== system ipad2/relay8c ==
  note: ic8
  Current Measurement : powerlib/Measurements/Current Measurement  PhasorSimulation=off  OutputType=Complex  PSBequivalent=0
  Scope : Scope
      settings: SaveName=ScopeData22
  To Workspace : ToWorkspace  VariableName=ic8  SampleTime=1/1600  SaveFormat=Array
  Conn1 : PMIOPort  Port=1  Side=Left
  Conn2 : PMIOPort  Port=2  Side=Right
  wires:
  Current Measurement/1 -> To Workspace/1, Scope/1
  connections:
  Conn2/RConn1 -- Current Measurement/RConn1
  Conn1/RConn1 -- Current Measurement/LConn1

== system ipad2/relay9a ==
  Current Measurement : powerlib/Measurements/Current Measurement  PhasorSimulation=off  OutputType=Complex  PSBequivalent=0
  Display : Display
  Scope : Scope
      settings: SaveName=ScopeData23
  ia9 : ToWorkspace  VariableName=ia9  SampleTime=1/1600  SaveFormat=Array
  Conn1 : PMIOPort  Port=1  Side=Left
  Conn2 : PMIOPort  Port=2  Side=Right
  wires:
  Current Measurement/1 -> ia9/1, Scope/1, Display/1
  connections:
  Conn1/RConn1 -- Current Measurement/LConn1
  Conn2/RConn1 -- Current Measurement/RConn1

== system ipad2/relay9b ==
  Current Measurement : powerlib/Measurements/Current Measurement  PhasorSimulation=off  OutputType=Complex  PSBequivalent=0
  Scope : Scope
      settings: SaveName=ScopeData24
  ib9 : ToWorkspace  VariableName=ib9  SampleTime=1/1600  SaveFormat=Array
  Conn1 : PMIOPort  Port=1  Side=Left
  Conn2 : PMIOPort  Port=2  Side=Right
  wires:
  Current Measurement/1 -> ib9/1, Scope/1
  connections:
  Conn2/RConn1 -- Current Measurement/RConn1
  Conn1/RConn1 -- Current Measurement/LConn1

== system ipad2/relay9c ==
  Current Measurement : powerlib/Measurements/Current Measurement  PhasorSimulation=off  OutputType=Complex  PSBequivalent=0
  Scope : Scope
      settings: SaveName=ScopeData25
  ic9 : ToWorkspace  VariableName=ic9  SampleTime=1/1600  SaveFormat=Array
  Conn1 : PMIOPort  Port=1  Side=Left
  Conn2 : PMIOPort  Port=2  Side=Right
  wires:
  Current Measurement/1 -> ic9/1, Scope/1
  connections:
  Conn1/RConn1 -- Current Measurement/LConn1
  Conn2/RConn1 -- Current Measurement/RConn1
